simulink model "BMSController"  (R2024b)
settings: configuration reference "VehicleFixed100ms" (kept outside this file)
undefined symbols (not defined in the file): PlntBattNumCellSer, PlntBattTempInitDegC
settings Model: DataDictionary=VirtualVehicleTemplate.sldd  ModifiedByFormat=The MathWorks, Inc.  PauseTimes=0  ExtModeTrigDuration=5  Creator=The MathWorks, Inc.  LastModifiedBy=The MathWorks, Inc.
settings ConfigSetRef: SourceName=VehicleFixed100ms

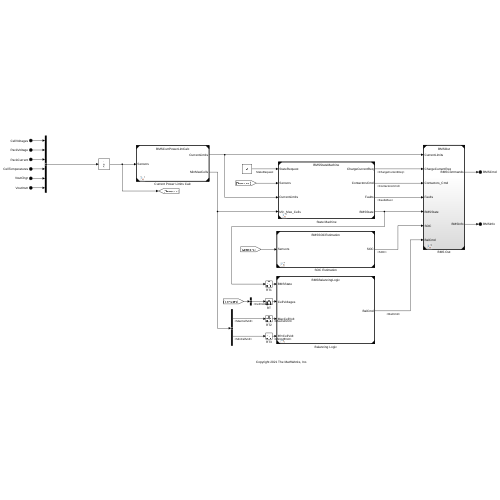
[thumbnail: Simulink's stored preview of the top-level diagram]
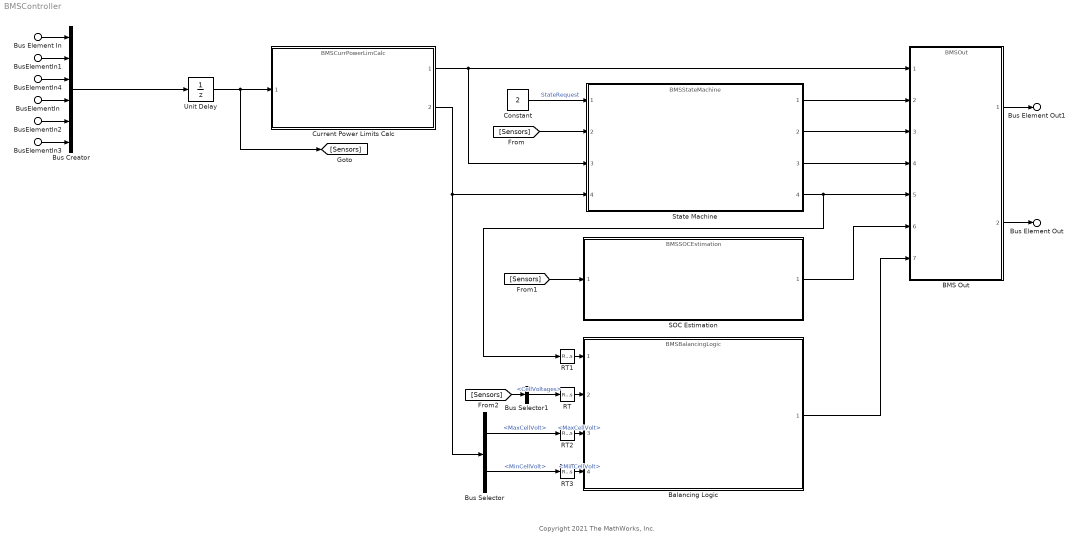
== system BMSController ==
  note: Copyright 2021 The MathWorks, Inc.
  Bus Element In : Inport  PortName=BMSSensors  Element=CellVoltages
  BusElementIn : Inport  PortName=BMSSensors  Element=CellTemperatures
  BusElementIn1 : Inport  PortName=BMSSensors  Element=PackVoltage
  BusElementIn2 : Inport  PortName=BMSSensors  Element=VoutChgr
  BusElementIn3 : Inport  PortName=BMSSensors  Element=VoutInvtr
  BusElementIn4 : Inport  PortName=BMSSensors  Element=PackCurrent
  BMS Out : ModelReference  ModelNameDialog=BMSOut.slx  ModelReferenceVersion=9.1
  Balancing Logic : ModelReference  ModelNameDialog=BMSBalancingLogic.slx  ModelReferenceVersion=9.4
  Bus Creator : BusCreator  Inputs=6
  Bus Selector : BusSelector  OutputSignals=MaxCellVolt,MinCellVolt
  Bus Selector1 : BusSelector  OutputSignals=CellVoltages
  Constant : Constant  Value=2  OutDataTypeStr=single  SampleTime=-1
  Current Power Limits Calc : ModelReference  ModelNameDialog=BMSCurrPowerLimCalc.slx  ModelReferenceVersion=9.2
  RT : RateTransition  InitialCondition=3.6*ones(1, PlntBattNumCellSer)
  RT1 : RateTransition  InitialCondition=single(0)  OutPortSampleTime=5
  RT2 : RateTransition  InitialCondition=single(3.6)  OutPortSampleTime=5
  RT3 : RateTransition  InitialCondition=single(3.6)  OutPortSampleTime=5
  SOC Estimation : ModelReference  ModelNameDialog=BMSSOCEstimation.slx  ModelReferenceVersion=9.1
  State Machine : ModelReference  ModelNameDialog=BMSStateMachine.slx  ModelReferenceVersion=9.1
  Unit Delay : UnitDelay  InitialCondition=struct('CellVoltages',3.6*ones(1, PlntBattNumCellSer),'PackVoltage',3.6*PlntBattNumCellSer,'PackCurrent',0,'CellTemperatures',PlntBattTempInitDegC*ones(1,PlntBattNumCellSer),'VoutChgr',0,'VoutInvtr',0)  SampleTime=-1  HasFrameUpgradeWarning=on
  Bus Element Out : Outport  PortName=BMSInfo
  Bus Element Out1 : Outport  Port=2  PortName=BMSCmd
  wires:
  State Machine/4 -> BMS Out/5, RT1/1
  Constant/1 -> State Machine/1  "StateRequest"
  Bus Selector1/1 -> RT/1  "<CellVoltages>"
  SOC Estimation/1 -> BMS Out/6
  Balancing Logic/1 -> BMS Out/7
  BMS Out/1 -> Bus Element Out1/1
  BMS Out/2 -> Bus Element Out/1
  Current Power Limits Calc/1 -> State Machine/3, BMS Out/1
  State Machine/2 -> BMS Out/3
  State Machine/1 -> BMS Out/2
  State Machine/3 -> BMS Out/4
  [Sensors] -> State Machine/2
  RT/1 -> Balancing Logic/2
  RT1/1 -> Balancing Logic/1
  Current Power Limits Calc/2 -> Bus Selector/1, State Machine/4
  Bus Selector/1 -> RT2/1  "<MaxCellVolt>"
  Bus Selector/2 -> RT3/1  "<MinCellVolt>"
  RT2/1 -> Balancing Logic/3  "<MaxCellVolt>"
  RT3/1 -> Balancing Logic/4  "<MinCellVolt>"
  [Sensors] -> Bus Selector1/1
  Unit Delay/1 -> [Sensors], Current Power Limits Calc/1
  BusElementIn2/1 -> Bus Creator/5
  BusElementIn/1 -> Bus Creator/4
  Bus Element In/1 -> Bus Creator/1
  BusElementIn1/1 -> Bus Creator/2
  BusElementIn3/1 -> Bus Creator/6
  BusElementIn4/1 -> Bus Creator/3
  Bus Creator/1 -> Unit Delay/1
  [Sensors] -> SOC Estimation/1
